simulink model "SEGWAY_SIM_SFR"  (R2021b)
settings: Solver=ode23t  StartTime=0.0  StopTime=10  FixedStep=ts  MaxStep=ts  RelTol=1e-6  AbsTol=1e-9
values from neighbouring files (symbols this model uses):
  alfa1 = 0.8    [CONTROL_SEGWAY.m]    (also in Control_Segway_2015.m; ensayo1.mat; ensayo2_wn4.8_seta_0.7.mat; ensayo3_wn5.3_seta_0.55.mat)
  g = 9.81    [CONTROL_SEGWAY.m]    (also in Control_Segway_2015.m; ensayo1.mat; ensayo2_wn4.8_seta_0.7.mat; ensayo3_wn5.3_seta_0.55.mat)
  h = 0.073    [CONTROL_SEGWAY.m]    (also in Control_Segway_2015.m; ensayo1.mat; ensayo2_wn4.8_seta_0.7.mat; ensayo3_wn5.3_seta_0.55.mat)
  Kcd = Ka(1, 1:3)    [Control_Segway_2015.m]    (also in ensayo1.mat = [-68.2484140277 -10.6212069049 -81.1609824123]; ensayo2_wn4.8_seta_0.7.mat = [-20.5032172519 -3.21085847646 -25.3008871114]; ensayo3_wn5.3_seta_0.55.mat = [-22.2986458352 -3.45646199395 -23.8255259596]; ensayo3_wn5.5_seta_0.7.mat = [-22.2599657852 -3.62971388524 -28.5561648788])
  param = [M m Ith Imr h W R Ke Rm Trmax Dm n]    [CONTROL_SEGWAY.m]    (also in Control_Segway_2015.m; ensayo1.mat = [0.6 0.034 0.001425 0.0037532 0.073 0.15 0.0408 0.01 4.5 0 0; ensayo2_wn4.8_seta_0.7.mat = [0.6 0.034 0.001425 0.0037532 0.073 0.15 0.0408 0.01 4.5 0 0; ensayo3_wn5.3_seta_0.55.mat = [0.6 0.034 0.001425 0.0037532 0.073 0.15 0.0408 0.01 4.5 0 0)
  R = 81.6e-3/2    (= 0.0408)    [CONTROL_SEGWAY.m]    (also in Control_Segway_2015.m; ensayo1.mat; ensayo2_wn4.8_seta_0.7.mat; ensayo3_wn5.3_seta_0.55.mat)
  ts = 5e-3    (= 0.005)    [CONTROL_SEGWAY.m]    (also in Control_Segway_2015.m; ensayo1.mat; ensayo2_wn4.8_seta_0.7.mat; ensayo3_wn5.3_seta_0.55.mat)
  X0 = [0, 0, th0*pi/180]'    [Control_Segway_2015.m]
settings Model: Creator=zamora  LastModifiedBy=ferna
settings SolverCC: AutoScaleAbsTol=off  ZeroCrossControl=EnableAll  ZeroCrossAlgorithm=Adaptive  AlgebraicLoopSolver=TrustRegion
settings DataIOCC: SaveFormat=Array  SignalLoggingSaveFormat=ModelDataLogs  SaveOutput=off  SaveTime=off  ReturnWorkspaceOutputs=off  StateSaveName=x  TimeSaveName=t  OutputSaveName=y
settings OptimizationCC: BlockReduction=off  BooleanDataType=off  DefaultParameterBehavior=Inlined  BufferReuse=off  ExpressionDepthLimit=2147483647  LifeSpan=inf
settings DebuggingCC: SaveWithParameterizedLinksMsg=none  UnderspecifiedInitializationDetection=Classic  MergeDetectMultiDrivingBlocksExec=none  SignalResolutionControl=TryResolveAllWithWarning  MaxConsecutiveZCsMsg=none  IgnoredZcDiagnostic=none  MultiTaskDSMMsg=warning  MultiTaskCondExecSysMsg=none  FcnCallInpInsideContextMsg=warning  StateNameClashWarn=warning  SFUnexpectedBacktrackingDiag=warning  SFNoUnconditionalDefaultTransitionDiag=warning  SFExecutionAtInitializationDiag=none  SFMachineParentedDataDiag=warning  ArithmeticOperatorsInVariantConditions=warning
settings HardwareCC: ProdBitPerPointer=32  ProdBitPerSizeT=32  ProdBitPerPtrDiffT=32  ProdLargestAtomicFloat=None  ProdIntDivRoundTo=Undefined  ProdEndianess=Unspecified  ProdWordSize=32  ProdHWDeviceType=32-bit Generic  TargetUnknown=on
settings ModelReferenceCC: PropagateSignalLabelsOutOfModel=off
settings SFSimCC: SimUseLocalCustomCode=off  CustomCodeUndefinedFunction=UseInterfaceOnly
settings RTWCC: TemplateMakefile=grt_unix.tmf  RTWUseLocalCustomCode=off
settings CodeAppCC: StateflowObjectComments=on
settings GRTTargetCC: TargetLangStandard=C89/C90 (ANSI)  CombineOutputUpdateFcns=off  GRTInterface=on
settings ConfigComp: CovMetricSettings=dw  CovSaveCumulativeToWorkspaceVar=on  CovSaveSingleToWorkspaceVar=on  CovExternalEMLEnable=off  CovSFcnEnable=off

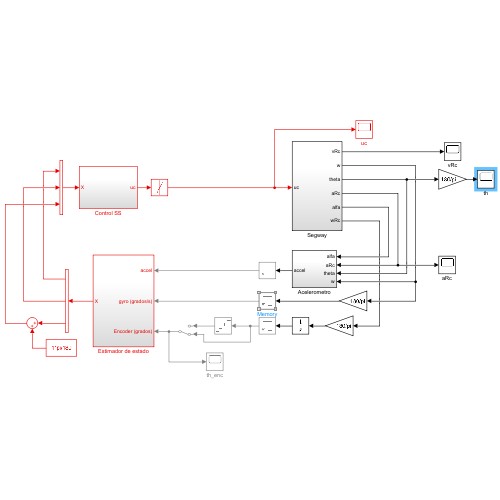
[thumbnail: Simulink's stored preview of the top-level diagram]
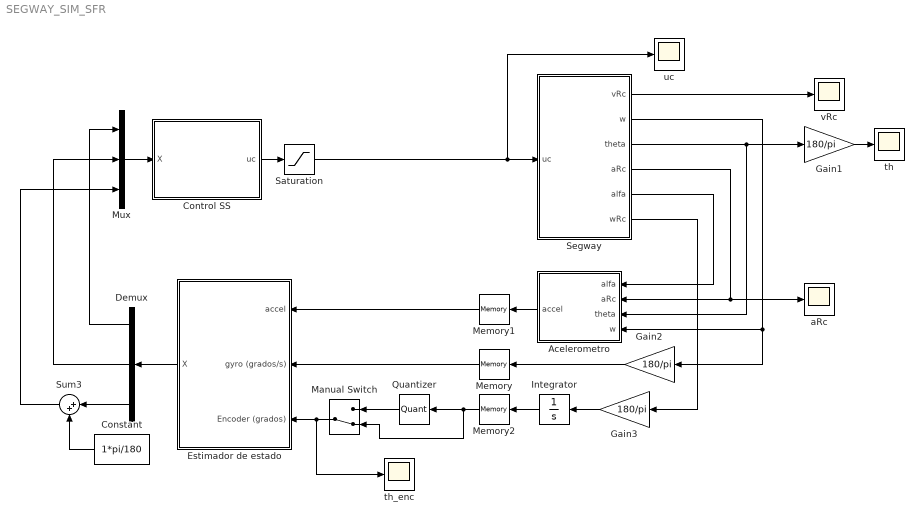
== system SEGWAY_SIM_SFR ==
  Acelerometro : Subsystem
  Constant : Constant  Value=1*pi/180  SampleTime=ts
  Control SS : Subsystem
  Demux : Demux  Outputs=3
  Estimador de estado : Subsystem
  Gain1 : Gain  Gain=180/pi
  Gain2 : Gain  Gain=180/pi
  Gain3 : Gain  Gain=180/pi
  Integrator : Integrator
  Manual Switch : ManualSwitch  CurrentSetting=0
  Memory : Memory
  Memory1 : Memory
  Memory2 : Memory
  Mux : Mux  Inputs=3
  Quantizer : Quantizer  QuantizationInterval=1
  Saturation : Saturate  UpperLimit=8.5  LowerLimit=-8.5
  Segway : Subsystem
  Sum3 : Sum  Inputs=|++
  aRc : Scope
  th : Scope
  th_enc : Scope
  uc : Scope
  vRc : Scope
  wires:
  Gain1/1 -> th/1
  Integrator/1 -> Memory2/1
  Segway/5(alfa) -> Acelerometro/1(alfa)
  Segway/4(aRc) -> aRc/1, Acelerometro/2(aRc)
  Segway/2(w) -> Gain2/1, Acelerometro/4(w)
  Segway/1(vRc) -> vRc/1
  Demux/2 -> Mux/2
  Sum3/1 -> Mux/3
  Gain2/1 -> Memory/1
  Gain3/1 -> Integrator/1
  Demux/3 -> Sum3/1
  Mux/1 -> Control SS/1(X)
  Demux/1 -> Mux/1
  Estimador de estado/1(X) -> Demux/1
  Acelerometro/1(accel) -> Memory1/1
  Control SS/1(uc) -> Saturation/1
  Segway/3(theta) -> Acelerometro/3(theta), Gain1/1
  Saturation/1 -> uc/1, Segway/1(uc)
  Memory1/1 -> Estimador de estado/1(accel)
  Memory/1 -> Estimador de estado/2(gyro (grados/s))
  Memory2/1 -> Manual Switch/2, Quantizer/1
  Manual Switch/1 -> Estimador de estado/3(Encoder (grados)), th_enc/1
  Quantizer/1 -> Manual Switch/1
  Constant/1 -> Sum3/2
  Segway/6(wRc) -> Gain3/1

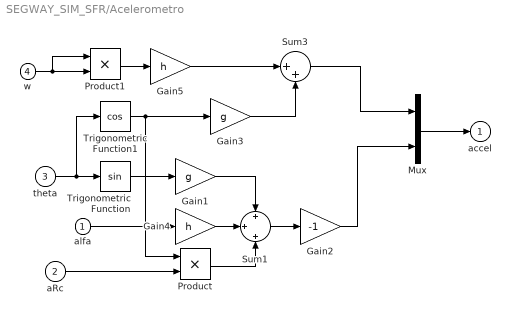
== system SEGWAY_SIM_SFR/Acelerometro ==
  alfa : Inport
  aRc : Inport  Port=2  SampleTime=0
  theta : Inport  Port=3  SampleTime=0
  w : Inport  Port=4
  Gain1 : Gain  Gain=g
  Gain2 : Gain  Gain=-1
  Gain3 : Gain  Gain=g
  Gain4 : Gain  Gain=h
  Gain5 : Gain  Gain=h
  Mux : Mux  Inputs=2
  Product : Product
  Product1 : Product
  Sum1 : Sum  Inputs=+|+|+
  Sum3 : Sum  Inputs=|++
  Trigonometric Function : Trigonometry
  Trigonometric Function1 : Trigonometry  Operator=cos
  accel : Outport  InitialOutput=0  VectorParamsAs1DForOutWhenUnconnected=off
  wires:
  Gain3/1 -> Sum3/2
  Gain5/1 -> Sum3/1
  Mux/1 -> accel/1
  Product1/1 -> Gain5/1
  alfa/1 -> Gain4/1
  w/1 -> Product1/1, Product1/2
  Sum3/1 -> Mux/1
  Sum1/1 -> Gain2/1
  Gain4/1 -> Sum1/2
  Gain1/1 -> Sum1/1
  theta/1 -> Trigonometric Function1/1, Trigonometric Function/1
  Gain2/1 -> Mux/2
  Trigonometric Function/1 -> Gain1/1
  Trigonometric Function1/1 -> Product/1, Gain3/1
  aRc/1 -> Product/2
  Product/1 -> Sum1/3

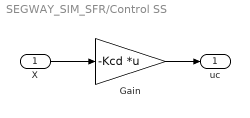
== system SEGWAY_SIM_SFR/Control SS ==
  X : Inport  SampleTime=ts
  Gain : Gain  Gain=-Kcd  Multiplication=Matrix(K*u)
  uc : Outport  VectorParamsAs1DForOutWhenUnconnected=off
  wires:
  Gain/1 -> uc/1
  X/1 -> Gain/1

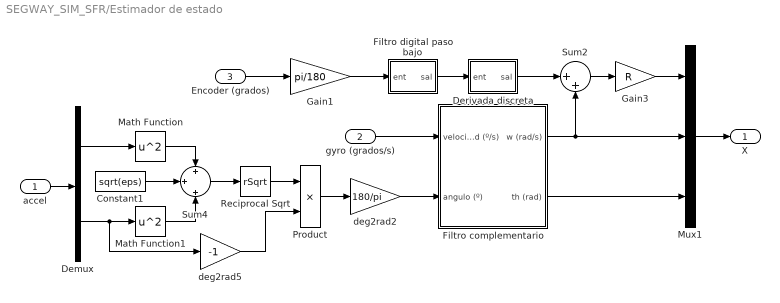
== system SEGWAY_SIM_SFR/Estimador de estado ==
  accel : Inport  SampleTime=ts
  gyro (grados/s) : Inport  Port=2  SampleTime=ts
  Encoder (grados) : Inport  Port=3  SampleTime=ts
  Constant1 : Constant  Value=sqrt(eps)  SampleTime=ts
  Demux : Demux  Outputs=2
  Derivada discreta : Subsystem  mask{ts=ts, opcion=Derivada en adelanto s=(1-z^-1)/ts}
      mask prompts: ts "Período de muestreo"; opcion "Método de discretización"
      mask init:
      | z=tf('z',ts);
      | switch(opcion)
      |     case 1
      |         derivada=minreal((1-z^-1)/ts);
      |     case 2
      |         derivada=minreal(2*(1-z^-1)/ts/(1+z^-1));
      |     case 3
      |         derivada=minreal((1.5-2*z^-1+0.5*z^-2)/ts);
      | end
      mask TypeOptions opcion: Derivada en adelanto s=(1-z^-1)/ts  | Trapezoidal s=2*(1-z^-1)/ts/(1+z^-1) | Derivada por aproximación parabólica s=(1.5-2*z^-1+0.5z^-2)/ts
  Filtro complementario : Subsystem
  Filtro digital paso bajo : Subsystem  mask{alfa=alfa1, x0=0, ts=ts}
      mask prompts: alfa "Constante de filtrado"; x0 "Condición inicial"; ts "Período de muestreo"
  Gain1 : Gain  Gain=pi/180  OutDataTypeStr=Inherit: Same as input  ParamDataTypeStr=Inherit: Same as input
  Gain3 : Gain  Gain=R  OutDataTypeStr=Inherit: Same as input  ParamDataTypeStr=Inherit: Same as input
  Math Function : Math  Operator=square  SignedPower=on  SaturateOnIntegerOverflow=on
  Math Function1 : Math  Operator=square  SignedPower=on  SaturateOnIntegerOverflow=on
  Mux1 : Mux  Inputs=3
  Product : Product
  Reciprocal Sqrt : Sqrt  Operator=rSqrt  SaturateOnIntegerOverflow=on
  Sum2 : Sum  Inputs=|++  OutDataTypeStr=Inherit: Same as first input
  Sum4 : Sum  Inputs=+|+|+
  deg2rad2 : Gain  Gain=180/pi  OutDataTypeStr=Inherit: Same as input  ParamDataTypeStr=Inherit: Same as input
  deg2rad5 : Gain  Gain=-1  OutDataTypeStr=Inherit: Same as input  ParamDataTypeStr=Inherit: Same as input
  X : Outport  VectorParamsAs1DForOutWhenUnconnected=off
  wires:
  gyro (grados/s)/1 -> Filtro complementario/1(velocidad (º/s))
  Sum2/1 -> Gain3/1
  Mux1/1 -> X/1
  Encoder (grados)/1 -> Gain1/1
  Gain3/1 -> Mux1/1
  Filtro complementario/1(w (rad/s)) -> Sum2/2, Mux1/2
  Filtro complementario/2(th (rad)) -> Mux1/3
  Product/1 -> deg2rad2/1
  deg2rad2/1 -> Filtro complementario/2(angulo (º))
  accel/1 -> Demux/1
  Demux/1 -> Math Function/1
  Math Function/1 -> Sum4/1
  Sum4/1 -> Reciprocal Sqrt/1
  Demux/2 -> deg2rad5/1, Math Function1/1
  deg2rad5/1 -> Product/2
  Filtro digital paso bajo/1(sal) -> Derivada discreta/1(ent)
  Derivada discreta/1(sal) -> Sum2/1
  Gain1/1 -> Filtro digital paso bajo/1(ent)
  Reciprocal Sqrt/1 -> Product/1
  Math Function1/1 -> Sum4/3
  Constant1/1 -> Sum4/2

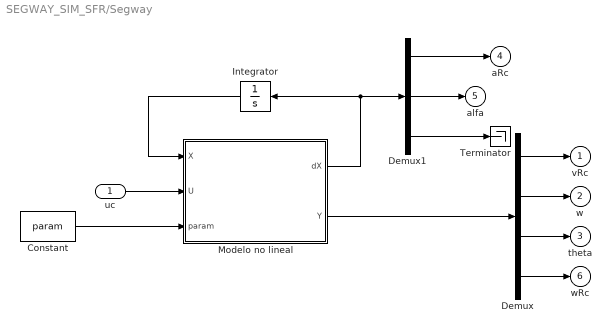
== system SEGWAY_SIM_SFR/Segway ==
  uc : Inport  SampleTime=0
  Constant : Constant  Value=param  SampleTime=0
  Demux : Demux
  Demux1 : Demux  Outputs=3
  Integrator : Integrator  InitialCondition=X0
  Modelo no lineal : MATLAB Function  TreatAsAtomicUnit=on
  Terminator : Terminator
  vRc : Outport  InitialOutput=0  VectorParamsAs1DForOutWhenUnconnected=off
  w : Outport  Port=2  InitialOutput=0  VectorParamsAs1DForOutWhenUnconnected=off
  theta : Outport  Port=3  InitialOutput=0  VectorParamsAs1DForOutWhenUnconnected=off
  aRc : Outport  Port=4  InitialOutput=0  VectorParamsAs1DForOutWhenUnconnected=off
  alfa : Outport  Port=5  InitialOutput=0  VectorParamsAs1DForOutWhenUnconnected=off
  wRc : Outport  Port=6  InitialOutput=0  VectorParamsAs1DForOutWhenUnconnected=off
  wires:
  Modelo no lineal/1(dX) -> Demux1/1, Integrator/1
  Integrator/1 -> Modelo no lineal/1(X)
  Constant/1 -> Modelo no lineal/3(param)
  uc/1 -> Modelo no lineal/2(U)
  Demux/1 -> vRc/1
  Demux/2 -> w/1
  Demux/3 -> theta/1
  Modelo no lineal/2(Y) -> Demux/1
  Demux1/2 -> alfa/1
  Demux1/3 -> Terminator/1
  Demux1/1 -> aRc/1
  Demux/4 -> wRc/1

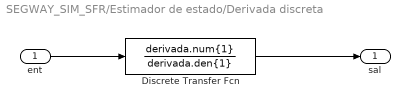
== system SEGWAY_SIM_SFR/Estimador de estado/Derivada discreta ==
  ent : Inport  SampleTime=ts
  Discrete Transfer Fcn : DiscreteTransferFcn  Numerator=derivada.num{1}  Denominator=derivada.den{1}
  sal : Outport  VectorParamsAs1DForOutWhenUnconnected=off
  wires:
  ent/1 -> Discrete Transfer Fcn/1
  Discrete Transfer Fcn/1 -> sal/1

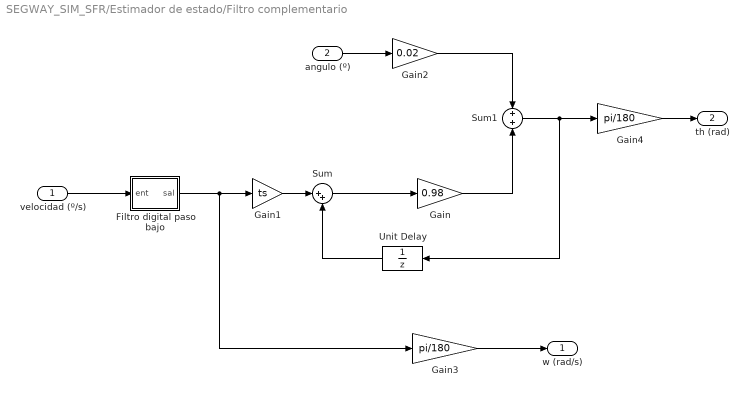
== system SEGWAY_SIM_SFR/Estimador de estado/Filtro complementario ==
  velocidad (º/s) : Inport  SampleTime=ts
  angulo (º) : Inport  Port=2  SampleTime=ts
  Filtro digital paso bajo : Subsystem  mask{alfa=alfa1, x0=0, ts=ts}
      mask prompts: alfa "Constante de filtrado"; x0 "Condición inicial"; ts "Período de muestreo"
  Gain : Gain  Gain=0.98
  Gain1 : Gain  Gain=ts
  Gain2 : Gain  Gain=0.02
  Gain3 : Gain  Gain=pi/180
  Gain4 : Gain  Gain=pi/180
  Sum : Sum  Inputs=|++
  Sum1 : Sum  Inputs=+|+
  Unit Delay : UnitDelay  SampleTime=-1  HasFrameUpgradeWarning=on
  w (rad/s) : Outport  VectorParamsAs1DForOutWhenUnconnected=off
  th (rad) : Outport  Port=2  VectorParamsAs1DForOutWhenUnconnected=off
  wires:
  Gain1/1 -> Sum/1
  Unit Delay/1 -> Sum/2
  Sum/1 -> Gain/1
  Gain/1 -> Sum1/2
  angulo (º)/1 -> Gain2/1
  Gain2/1 -> Sum1/1
  Sum1/1 -> Gain4/1, Unit Delay/1
  Gain3/1 -> w (rad/s)/1
  Gain4/1 -> th (rad)/1
  velocidad (º/s)/1 -> Filtro digital paso bajo/1(ent)
  Filtro digital paso bajo/1(sal) -> Gain3/1, Gain1/1

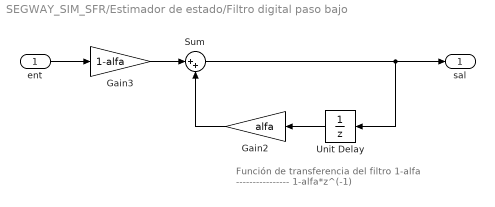
== system SEGWAY_SIM_SFR/Estimador de estado/Filtro digital paso bajo ==
  note: Función de transferencia del filtro
      |                        1-alfa
      |                  ----------------
      |                   1-alfa*z^(-1)
  ent : Inport  SampleTime=ts
  Gain2 : Gain  Gain=alfa  OutDataTypeStr=Inherit: Same as input  ParamDataTypeStr=Inherit: Same as input
  Gain3 : Gain  Gain=1-alfa  OutDataTypeStr=Inherit: Same as input  ParamDataTypeStr=Inherit: Same as input
  Sum : Sum  Inputs=|++  OutDataTypeStr=Inherit: Same as first input
  Unit Delay : UnitDelay  SampleTime=-1  HasFrameUpgradeWarning=on
  sal : Outport  VectorParamsAs1DForOutWhenUnconnected=off
  wires:
  ent/1 -> Gain3/1
  Gain3/1 -> Sum/1
  Gain2/1 -> Sum/2
  Unit Delay/1 -> Gain2/1
  Sum/1 -> sal/1, Unit Delay/1

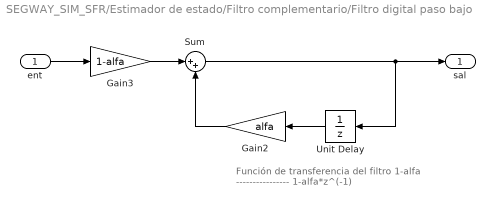
== system SEGWAY_SIM_SFR/Estimador de estado/Filtro complementario/Filtro digital paso bajo ==
  note: Función de transferencia del filtro
      |                        1-alfa
      |                  ----------------
      |                   1-alfa*z^(-1)
  ent : Inport  SampleTime=ts
  Gain2 : Gain  Gain=alfa  OutDataTypeStr=Inherit: Same as input  ParamDataTypeStr=Inherit: Same as input
  Gain3 : Gain  Gain=1-alfa  OutDataTypeStr=Inherit: Same as input  ParamDataTypeStr=Inherit: Same as input
  Sum : Sum  Inputs=|++  OutDataTypeStr=Inherit: Same as first input
  Unit Delay : UnitDelay  SampleTime=-1  HasFrameUpgradeWarning=on
  sal : Outport  VectorParamsAs1DForOutWhenUnconnected=off
  wires:
  Sum/1 -> Unit Delay/1, sal/1
  Unit Delay/1 -> Gain2/1
  Gain2/1 -> Sum/2
  Gain3/1 -> Sum/1
  ent/1 -> Gain3/1

== matlab function SEGWAY_SIM_SFR/Segway/Modelo no lineal ==
  data: X input; dX output; U input; param input; Y output
function [dX,Y] = segway(X,U,param)

%% Parametros
% Masa del chasis (kg)
M=param(1);
% Masa de la rueda incluyendo el rotor del motor (kg)
m=param(2);
% Momento de inercia de cabeceo del chasis (kg.m^2)
Ith=param(3);
% Momento de inercia del conjunto motor + rueda (kg.m^2)
Imr=param(4);
% Distancia al centro de gravedad del chasis medida desde el eje (m)
h=param(5);
% Distancia de separacion entre ruedas (m)
W=param(6);
% Radio de las rueda (m)
R=param(7);
% Constante electrica del motor (V.s/rad)
Ke=param(8);
% Constante mecanica del motor (N.m/A)
Kt=Ke;
% Resistencia electrica del motor
Rm=param(9);
% Par de friccion del motor (N.m) eje externo
Trmax=param(10);
% Coeficiente de friccion viscosa eje externo (N.m.s/rad)
Dm=param(11);
% Relacion de engranajes
n=param(12);


% Gravedad (m/s^2)
g=9.81;

%% Entradas
% Tension comun (V)
uc=U(1);

%% Variables de estado
% Velocidad comun lineal de las ruedas (m/s)
vRc=X(1);
% Velocidad angular de cabeceo (rad/s)
wth=X(2);
% Angulo de cabeceo (rad)
th=X(3);
% Velocidad angular de la rueda (rad/s)
wRc=vRc/R;
% Velocidad angular del motor
wmc=n*wRc-wth;


%% Motor
% Ecuacion electrica del motor
ic=(uc-Ke*wmc)/Rm;
% Par motor eje motor
Tmc=Kt*ic;
% Par motor límite (eje motor) para aplicación del par máximo de fricción (eje rueda)
wmc_aux = 5*[-2 -1 1 2];
Trc_aux = Trmax/n*[-1 -1 1 1];
% Tmc_lim=Tmc*(Tmc>-Trmax/n && Tmc<Trmax/n)-Trmax/n*(Tmc<=-Trmax/n)+Trmax*(Tmc>=Trmax/n);
% Par de friccion estatico (eje rueda)
% Trc=n*Tmc_lim*(abs(wmc)==0)+Trmax*sign(wmc)*(abs(wmc)>0);
Trc = interp1(wmc_aux,Trc_aux,wmc,'linear','extrap');
% Par neto (eje motor)
Tc=Tmc-Dm*wRc/n-Trc/n;

%% Avance del vehiculo y cabeceo
% 2*n*Tc/R = (2*(m+Imr/R^2)+M)*aRc + M*h*alfath*cos(th) - M*wth^2*h*sin(th)
% -2*Tc + M*g*h*sin(th) = M*h*cos(th)*aRc + (Ith+M*h^2)*alfath
% Se resuelve el sistema de ecuaciones anterior
matA_aux=[2*(m+Imr/R^2)+M   M*h*cos(th)
              M*h*cos(th)   Ith+M*h^2];
matB_aux=[2*n*Tc/R + M*wth^2*h*sin(th) ; -2*Tc + M*g*h*sin(th)];
aux=matA_aux\matB_aux;
aRc=aux(1);
alfath=aux(2); 

% Derivada del vector de estado
dX=[aRc alfath wth]';

%% Ecuaciones de salida
Y = [X; wRc];
